simulink model "Antenna_control"  (R2015a)
settings: Solver=ode45  StartTime=0.0  StopTime=10.0  RelTol=1e-3
settings Model: Creator=roman  LastModifiedBy=roman

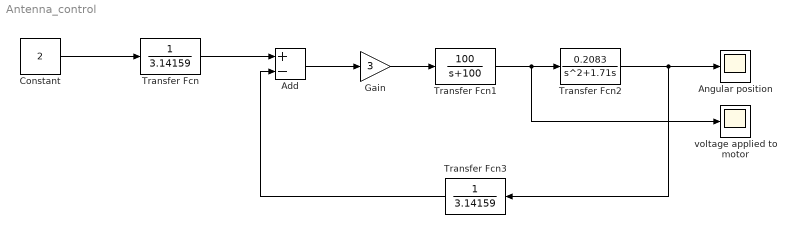
== system Antenna_control ==
  Add : Sum  Inputs=+-
  Angular position : Scope
      settings: TimeRange=30
  Constant : Constant  Value=2
  Gain : Gain  Gain=3
  Transfer Fcn : TransferFcn  Denominator=[3.14159]
  Transfer Fcn1 : TransferFcn  Numerator=[100]  Denominator=[1 100]
  Transfer Fcn2 : TransferFcn  Numerator=[0.2083]  Denominator=[1 1.71 0]
  Transfer Fcn3 : TransferFcn  Denominator=[3.14159]
  voltage applied to motor : Scope
      settings: TimeRange=20  YMin=0  YMax=2
  wires:
  Constant/1 -> Transfer Fcn/1
  Transfer Fcn/1 -> Add/1
  Add/1 -> Gain/1
  Gain/1 -> Transfer Fcn1/1
  Transfer Fcn1/1 -> voltage applied to motor/1, Transfer Fcn2/1
  Transfer Fcn2/1 -> Angular position/1, Transfer Fcn3/1
  Transfer Fcn3/1 -> Add/2
